simulink model "motor"  (R2017a)
settings: Solver=VariableStepAuto  StartTime=0.0  StopTime=10.0  RelTol=1e-3
settings Model: Creator=pedro  LastModifiedBy=pedro

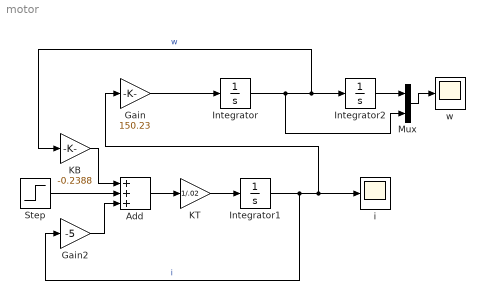
== system motor ==
  Add : Sum  Inputs=+++
  Gain : Gain  Gain=150.23
  Gain2 : Gain  Gain=-5
  Integrator : Integrator
  Integrator1 : Integrator
  Integrator2 : Integrator
  KB : Gain  Gain=-0.2388
  KT : Gain  Gain=1/.02
  Mux : Mux  Inputs=2
  Step : Step  SampleTime=0
  i : Scope
  w : Scope
  wires:
  Integrator/1 -> Mux/2, KB/1, Integrator2/1  "w"
  Integrator1/1 -> Gain2/1, i/1, Gain/1  "i"
  Gain/1 -> Integrator/1
  KB/1 -> Add/1
  Gain2/1 -> Add/3
  Step/1 -> Add/2
  Add/1 -> KT/1
  KT/1 -> Integrator1/1
  Integrator2/1 -> Mux/1
  Mux/1 -> w/1
